simulink library "LibWheels"  (R2019b)
settings: Solver=VariableStepAuto  StartTime=0.0  StopTime=10.0  RelTol=1e-3
undefined symbols (not defined in the file or in its folder): BrakeMaxPrs
libraries: VsrLibWheel x4
settings Model: Creator=9bt  LastModifiedBy=4qz

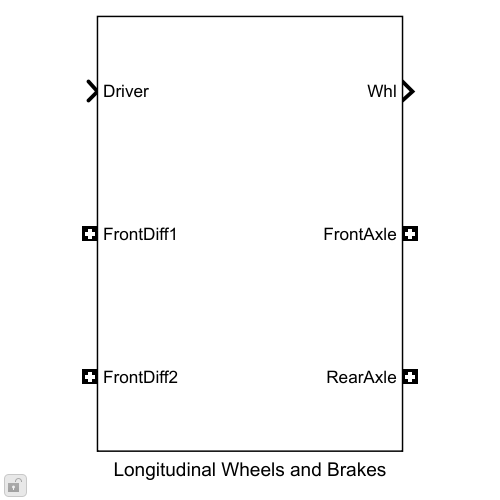
[thumbnail: Simulink's stored preview of the top-level diagram]
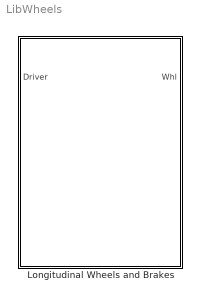
== system LibWheels ==
  Longitudinal Wheels and Brakes : Subsystem

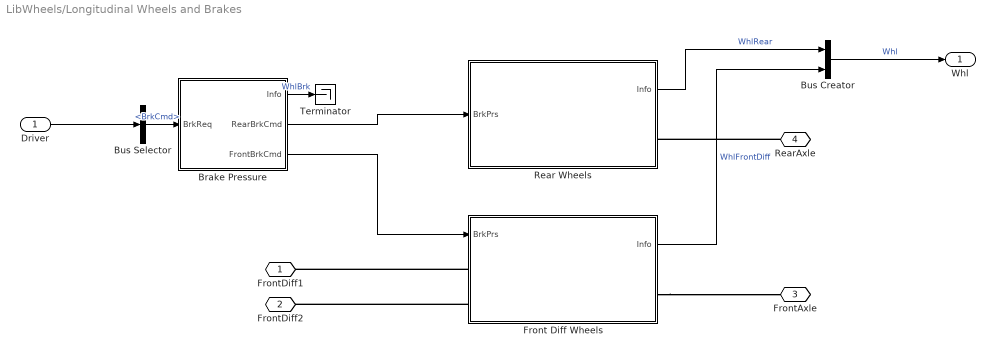
== system LibWheels/Longitudinal Wheels and Brakes ==
  Driver : Inport
  Brake Pressure : Subsystem
  Bus Creator : BusCreator  Inputs=2
  Bus Selector : BusSelector  OutputSignals=BrkCmd
  Front Diff Wheels : Subsystem
  Rear Wheels : Subsystem
  Terminator : Terminator
  FrontDiff1 : PMIOPort  Side=Left
  FrontDiff2 : PMIOPort  Port=2  Side=Left
  FrontAxle : PMIOPort  Port=3  Side=Right
  RearAxle : PMIOPort  Port=4  Side=Right
  Whl : Outport
  wires:
  Bus Creator/1 -> Whl/1  "Whl"
  Driver/1 -> Bus Selector/1
  Front Diff Wheels/1(Info) -> Bus Creator/2  "WhlFrontDiff"
  Rear Wheels/1(Info) -> Bus Creator/1  "WhlRear"
  Brake Pressure/1(Info) -> Terminator/1  "WhlBrk"
  Bus Selector/1 -> Brake Pressure/1(BrkReq)  "<BrkCmd>"
  Brake Pressure/2(RearBrkCmd) -> Rear Wheels/1(BrkPrs)
  Brake Pressure/3(FrontBrkCmd) -> Front Diff Wheels/1(BrkPrs)
  connections:
  Front Diff Wheels/LConn1 -- FrontDiff1/RConn1
  Front Diff Wheels/LConn2 -- FrontDiff2/RConn1
  Front Diff Wheels/RConn1 -- FrontAxle/RConn1
  RearAxle/RConn1 -- Rear Wheels/RConn1

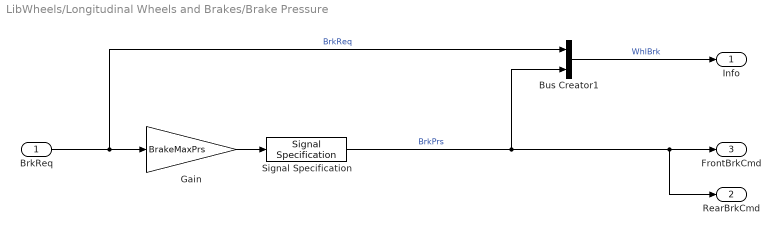
== system LibWheels/Longitudinal Wheels and Brakes/Brake Pressure ==
  BrkReq : Inport
  Bus Creator1 : BusCreator  Inputs=2
  Gain : Gain  Gain=BrakeMaxPrs
  Signal Specification : SignalSpecification  Unit=Pa
  Info : Outport
  RearBrkCmd : Outport  Port=2
  FrontBrkCmd : Outport  Port=3
  wires:
  Bus Creator1/1 -> Info/1  "WhlBrk"
  Signal Specification/1 -> Bus Creator1/2, RearBrkCmd/1, FrontBrkCmd/1  "BrkPrs"
  Gain/1 -> Signal Specification/1
  BrkReq/1 -> Bus Creator1/1, Gain/1  "BrkReq"

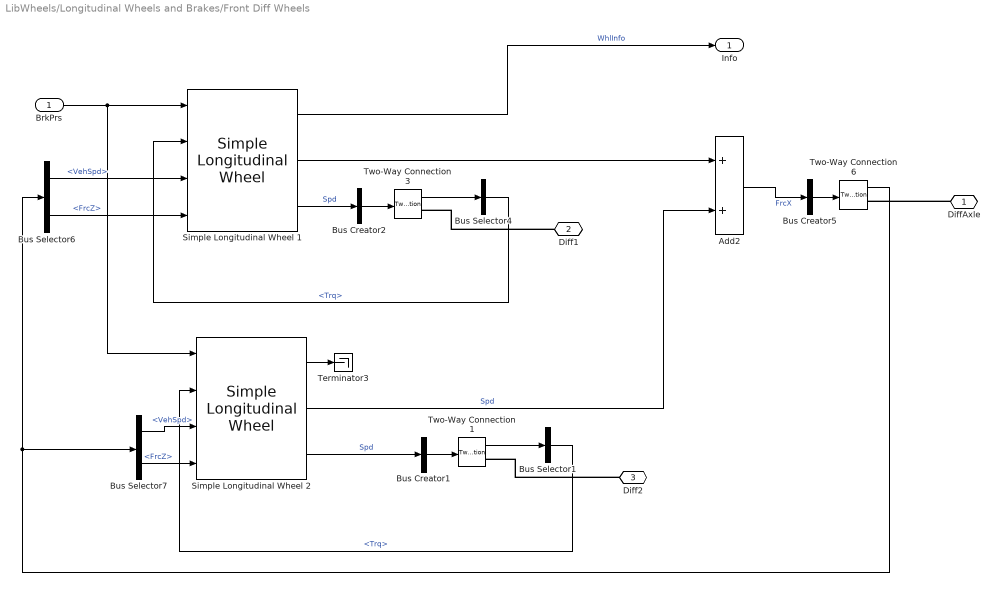
== system LibWheels/Longitudinal Wheels and Brakes/Front Diff Wheels ==
  BrkPrs : Inport
  Add2 : Sum
  Bus Creator1 : BusCreator  Inputs=1
  Bus Creator2 : BusCreator  Inputs=1
  Bus Creator5 : BusCreator  Inputs=1
  Bus Selector1 : BusSelector  OutputSignals=Trq
  Bus Selector4 : BusSelector  OutputSignals=Trq
  Bus Selector6 : BusSelector  OutputSignals=VehSpd,FrcZ
  Bus Selector7 : BusSelector  OutputSignals=VehSpd,FrcZ
  Simple Longitudinal Wheel 1 : VsrLibWheel/Simple Longitudinal Wheel  TireLoadedRadius=WhlRearLoadedRadius  C_rr=WhlRollingResistCnst  MaxBrkTrq=BrakeMaxTrq  MaxBrkPrs=BrakeMaxPrs  w_thresh=WhlSimVelTol
  Simple Longitudinal Wheel 2 : VsrLibWheel/Simple Longitudinal Wheel  TireLoadedRadius=WhlRearLoadedRadius  C_rr=WhlRollingResistCnst  MaxBrkTrq=BrakeMaxTrq  MaxBrkPrs=BrakeMaxPrs  w_thresh=WhlSimVelTol
  Terminator3 : Terminator
  Two-Way Connection1 : TwoWayConnection
  Two-Way Connection3 : TwoWayConnection
  Two-Way Connection6 : TwoWayConnection
  DiffAxle : PMIOPort  Side=Right
  Diff1 : PMIOPort  Port=2  Side=Left
  Diff2 : PMIOPort  Port=3  Side=Left
  Info : Outport
  wires:
  Simple Longitudinal Wheel 2/1 -> Terminator3/1
  Simple Longitudinal Wheel 1/1 -> Info/1  "WhlInfo"
  Bus Creator5/1 -> Two-Way Connection6/1
  Simple Longitudinal Wheel 2/2 -> Add2/2  "Spd"
  Add2/1 -> Bus Creator5/1  "FrcX"
  Two-Way Connection6/1 -> Bus Selector6/1, Bus Selector7/1
  Bus Selector7/2 -> Simple Longitudinal Wheel 2/4  "<FrcZ>"
  Bus Selector6/1 -> Simple Longitudinal Wheel 1/3  "<VehSpd>"
  Bus Selector7/1 -> Simple Longitudinal Wheel 2/3  "<VehSpd>"
  Simple Longitudinal Wheel 1/2 -> Add2/1
  BrkPrs/1 -> Simple Longitudinal Wheel 1/1, Simple Longitudinal Wheel 2/1
  Bus Selector6/2 -> Simple Longitudinal Wheel 1/4  "<FrcZ>"
  Bus Creator2/1 -> Two-Way Connection3/1
  Two-Way Connection3/1 -> Bus Selector4/1
  Bus Selector4/1 -> Simple Longitudinal Wheel 1/2  "<Trq>"
  Simple Longitudinal Wheel 1/3 -> Bus Creator2/1  "Spd"
  Bus Selector1/1 -> Simple Longitudinal Wheel 2/2  "<Trq>"
  Two-Way Connection1/1 -> Bus Selector1/1
  Bus Creator1/1 -> Two-Way Connection1/1
  Simple Longitudinal Wheel 2/3 -> Bus Creator1/1  "Spd"
  connections:
  DiffAxle/RConn1 -- Two-Way Connection6/RConn1
  Diff1/RConn1 -- Two-Way Connection3/RConn1
  Diff2/RConn1 -- Two-Way Connection1/RConn1

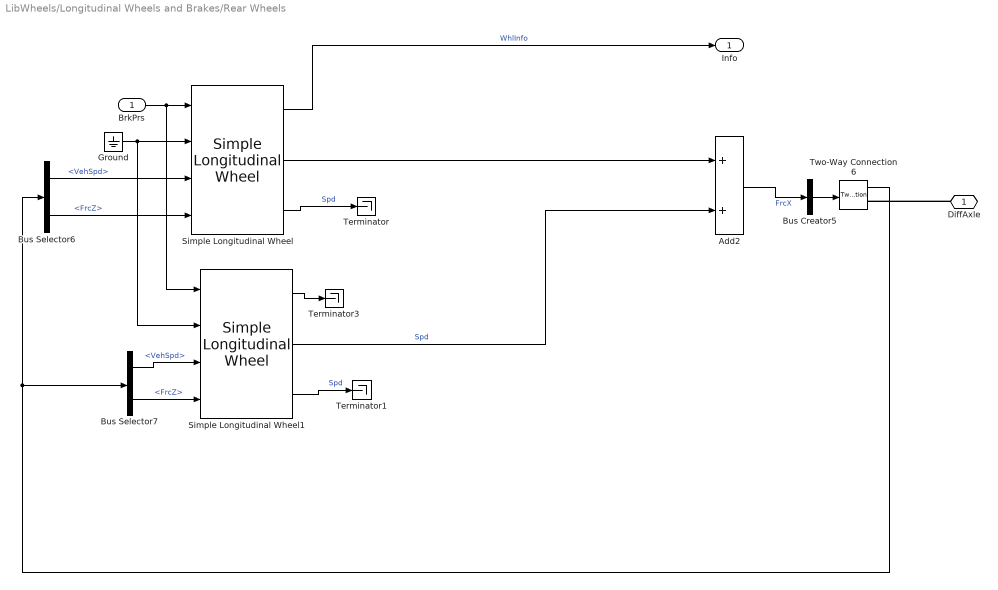
== system LibWheels/Longitudinal Wheels and Brakes/Rear Wheels ==
  BrkPrs : Inport
  Add2 : Sum
  Bus Creator5 : BusCreator  Inputs=1
  Bus Selector6 : BusSelector  OutputSignals=VehSpd,FrcZ
  Bus Selector7 : BusSelector  OutputSignals=VehSpd,FrcZ
  Ground : Ground
  Simple Longitudinal Wheel : VsrLibWheel/Simple Longitudinal Wheel  TireLoadedRadius=WhlFrontLoadedRadius  C_rr=WhlRollingResistCnst  MaxBrkTrq=BrakeMaxTrq  MaxBrkPrs=BrakeMaxPrs  w_thresh=WhlSimVelTol
  Simple Longitudinal Wheel1 : VsrLibWheel/Simple Longitudinal Wheel  TireLoadedRadius=WhlFrontLoadedRadius  C_rr=WhlRollingResistCnst  MaxBrkTrq=BrakeMaxTrq  MaxBrkPrs=BrakeMaxPrs  w_thresh=WhlSimVelTol
  Terminator : Terminator
  Terminator1 : Terminator
  Terminator3 : Terminator
  Two-Way Connection6 : TwoWayConnection
  DiffAxle : PMIOPort  Side=Right
  Info : Outport
  wires:
  Bus Selector6/2 -> Simple Longitudinal Wheel/4  "<FrcZ>"
  BrkPrs/1 -> Simple Longitudinal Wheel1/1, Simple Longitudinal Wheel/1
  Simple Longitudinal Wheel/2 -> Add2/1
  Bus Selector7/1 -> Simple Longitudinal Wheel1/3  "<VehSpd>"
  Bus Selector6/1 -> Simple Longitudinal Wheel/3  "<VehSpd>"
  Bus Selector7/2 -> Simple Longitudinal Wheel1/4  "<FrcZ>"
  Two-Way Connection6/1 -> Bus Selector6/1, Bus Selector7/1
  Add2/1 -> Bus Creator5/1  "FrcX"
  Simple Longitudinal Wheel1/2 -> Add2/2  "Spd"
  Bus Creator5/1 -> Two-Way Connection6/1
  Simple Longitudinal Wheel/3 -> Terminator/1  "Spd"
  Ground/1 -> Simple Longitudinal Wheel1/2, Simple Longitudinal Wheel/2
  Simple Longitudinal Wheel/1 -> Info/1  "WhlInfo"
  Simple Longitudinal Wheel1/3 -> Terminator1/1  "Spd"
  Simple Longitudinal Wheel1/1 -> Terminator3/1
  connections:
  DiffAxle/RConn1 -- Two-Way Connection6/RConn1
